simulink model "Buck_PI_DIGITAL_MG_PCD"  (R2024a)
settings: Solver=VariableStepAuto  StartTime=0.0  StopTime=1  RelTol=1e-3
libraries: spsSeriesRLCBranchLib x3, spsVoltageMeasurementLib x2, spsCurrentMeasurementLib x1, spsDiodeLib x1, spsDCVoltageSourceLib x1, spsGroundLib x1, spsMosfetLib x1, spsPWMGeneratorDCDCLib x1, sps_lib x1
settings Model: Creator=hardy  LastModifiedBy=marco
settings SolverCC: AlgebraicLoopSolver=TrustRegion
settings DebuggingCC: UnconnectedInputMsg=warning  UnconnectedOutputMsg=warning  UnconnectedLineMsg=warning
settings ModelReferenceCC: EnableRefExpFcnMdlSchedulingChecks=on
settings RTWCC: GPUComputeCapability=3.5

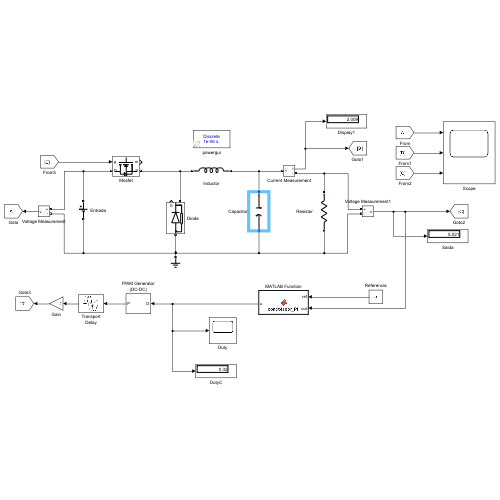
[thumbnail: Simulink's stored preview of the top-level diagram]
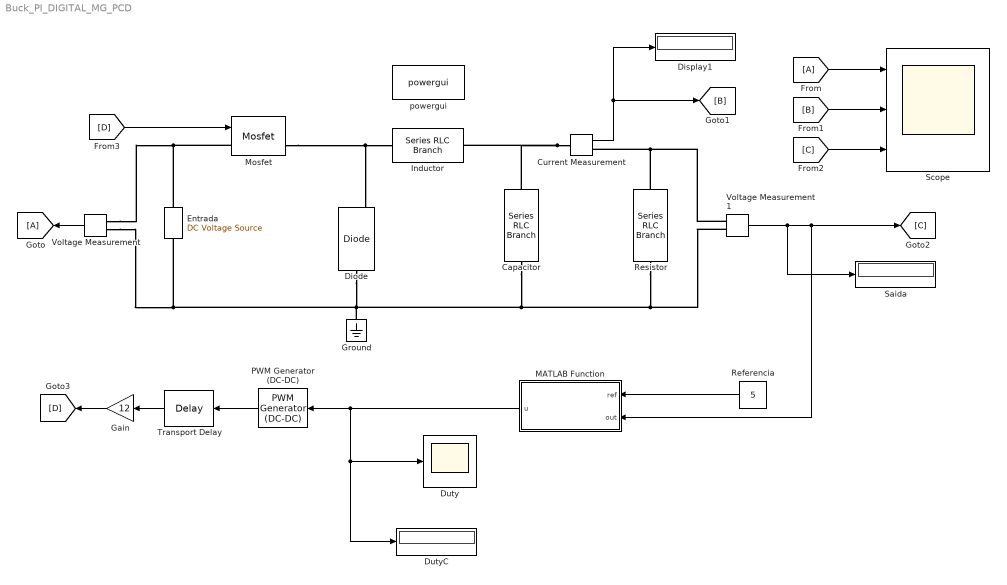
== system Buck_PI_DIGITAL_MG_PCD ==
  Capacitor : spsSeriesRLCBranchLib/Series RLC Branch  LConnTagsString=__new0  RConnTagsString=__new0  BranchType=C  Resistance=1  Inductance=1e-3  SetiL0=off  InitialCurrent=0  Capacitance=440e-6  Setx0=off  InitialVoltage=0  Measurements=None
  Current Measurement : spsCurrentMeasurementLib/Current Measurement  PhasorSimulation=off  OutputType=Complex  PSBequivalent=0
  Diode : spsDiodeLib/Diode  Ron=0.001  Lon=0  Vf=0  IC=0  UseSnubber=0  Rs=500  Cs=250e-9  Measurements=on
  Display1 : Display
  Duty : Scope
  DutyC : Display
  Entrada : spsDCVoltageSourceLib/DC Voltage Source  Amplitude=15  Measurements=None
  From : From
  Gain : Gain  Gain=12
  Goto : Goto
  Ground : spsGroundLib/Ground  LConnTagsString=a
  Inductor : spsSeriesRLCBranchLib/Series RLC Branch  LConnTagsString=__new0  RConnTagsString=__new0  BranchType=L  Resistance=1  Inductance=820e-6  SetiL0=off  InitialCurrent=0  Capacitance=1e-6  Setx0=off  InitialVoltage=0  Measurements=None
  MATLAB Function : MATLAB Function  TreatAsAtomicUnit=on
  Mosfet : spsMosfetLib/Mosfet  Ron=0.1  Lon=0  Rd=0.01  Vfd=0  IC=0  Rs=1e5  Cs=inf  Measurements=on
  PWM Generator (DC-DC) : spsPWMGeneratorDCDCLib/PWM Generator (DC-DC)  Fsw=60000  Ts=1e-6
  Referencia : Constant  Value=5
  Resistor : spsSeriesRLCBranchLib/Series RLC Branch  LConnTagsString=__new0  RConnTagsString=__new0  BranchType=R  Resistance=2.5  Inductance=1e-3  SetiL0=off  InitialCurrent=0  Capacitance=1e-6  Setx0=off  InitialVoltage=0  Measurements=None
  Saida : Display
  Scope : Scope  NumInputPorts=3
  Transport Delay : TransportDelay  DelayTime=100e-9
  Voltage Measurement : spsVoltageMeasurementLib/Voltage Measurement  PhasorSimulation=off  OutputType=Complex  PSBequivalent=0
  Voltage Measurement1 : spsVoltageMeasurementLib/Voltage Measurement  PhasorSimulation=off  OutputType=Complex  PSBequivalent=0
  powergui : sps_lib/powergui  Priority=1  SimulationMode=Discrete  SampleTime=1e-6  frequency=60  Iterations=50  frequencyindice=0  Pbase=100e6  ErrMax=1e-4  UnitsV=kV  UnitsW=MW  buscounter=0  FunctionMessages=off  echomessages=off  EnableUseOfTLC=off  CurrentSourceSwitches=off  DisableSnubberDevices=off  DisableRonSwitches=off  DisableVfSwitches=off  DisplayEquations=off  AutomaticDiscreteSolvers=off  SolverType=Tustin/Backward Euler (TBE)  Interpol=off  ExternalGateDelay=off  methode=off  Ts=100  x0status=blocks  SPID=on  SwTol=0  HookPort=off  NonlinearTolerance=1e-4  nMaxIteration=100  ContinueOnMaxIteration=off  RestoreLinks=warning  ResistiveCurrentMeasurement=off  Frange=[0:2:500]  Ylog=off  Xlog=on  ShowGrid=off  save=off  variable=ZData  structure=0  ZoomFFT=off  StartTime=0.0  cycles=1  DisplayStyle=1  fundamental=60  FreqAxis=off  MaxFrequency=1000  frequencyindicesteady=1  RmsSteady=1  display=off
  wires:
  Voltage Measurement/1 -> Goto/1
  Voltage Measurement1/1 -> MATLAB Function/2(out), [C], Saida/1
  From/1 -> Scope/1
  [B] -> Scope/2
  [C] -> Scope/3
  Current Measurement/1 -> Display1/1, [B]
  Referencia/1 -> MATLAB Function/1(ref)
  [D] -> Mosfet/1
  MATLAB Function/1(u) -> DutyC/1, Duty/1, PWM Generator (DC-DC)/1
  Gain/1 -> [D]
  PWM Generator (DC-DC)/1 -> Transport Delay/1
  Transport Delay/1 -> Gain/1
  connections:
  Entrada/RConn1 -- Mosfet/LConn1 -- Voltage Measurement/LConn1
  Mosfet/RConn1 -- Inductor/LConn1 -- Diode/RConn1
  Current Measurement/LConn1 -- Capacitor/LConn1 -- Inductor/RConn1
  Resistor/LConn1 -- Voltage Measurement1/LConn1 -- Current Measurement/RConn1
  Resistor/RConn1 -- Voltage Measurement1/LConn2 -- Capacitor/RConn1 -- Ground/LConn1 -- Diode/LConn1 -- Voltage Measurement/LConn2 -- Entrada/LConn1

== matlab function Buck_PI_DIGITAL_MG_PCD/MATLAB Function ==
  data: ref input; u output; out input
function u = controlador_PI(ref, out)
% Entradas:
%  ref - valor de referência (setpoint)
%  y   - valor de saída medido
% Saída:
%  u   - saída do controlador PI

% Parâmetros do controlador
Kp = 0.01;       % Ganho proporcional
Ki = 10;       % Ganho integral

% Persistência das variáveis
persistent integralErro
if isempty(integralErro)
    integralErro = 0;
end

% Cálculo do erro
erro = ref - out;

% Tempo de amostragem (ajuste conforme seu sistema)
Ts = 1e-6;

% Integração do erro
integralErro = integralErro + erro * Ts;

% Saída do controlador
u = Kp * erro + Ki * integralErro;
